simulink model "Satellite_Open_Loop_Model"  (R2018b)
settings: Solver=VariableStepAuto  StartTime=0.0  StopTime=200  RelTol=1e-3
values from neighbouring files (symbols this model uses):
  a = 0.5736    [Lab1.m]    (also in Micro_Sat_Open_Loop.m)
  J_r = 0.0004    [Lab1.m]    (also in Micro_Sat_Open_Loop.m)
  J_s = 31.38    [Lab1.m]    (also in Micro_Sat_Open_Loop.m)
  noise = 10^-9    (= 1e-09)    [Lab1.m]    (also in Micro_Sat_Open_Loop.m)
  T_d = 0.001    [Lab1.m]    (also in Micro_Sat_Open_Loop.m)
  T_e = 0.5    [Lab1.m]    (also in Micro_Sat_Open_Loop.m)
  Tc_max = 0.05    [Lab1.m]    (also in Micro_Sat_Open_Loop.m)
  To_m = 0.8    [Lab1.m]    (also in Micro_Sat_Open_Loop.m)
  w = 2.6268    [Lab1.m]    (also in Micro_Sat_Open_Loop.m)
  w_sat = wr_max*2*pi/60    (= 293.215314335)    [Micro_Sat_Open_Loop.m]
undefined symbols (not defined in the file or in its folder): sigbuilder_block
settings Model: Creator=Yavuz  LastModifiedBy=EKOCULU

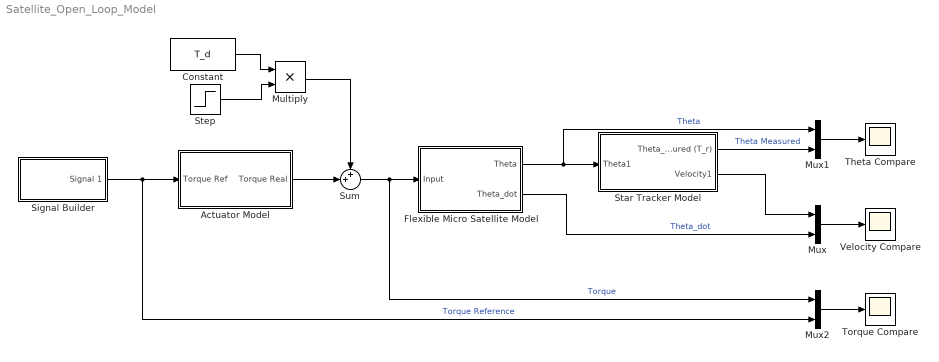
== system Satellite_Open_Loop_Model ==
  Actuator Model : Subsystem
  Constant : Constant  Value=T_d
  "Flexible Micro Satellite Model " : Subsystem
  Multiply : Product
  Mux : Mux  Inputs=2
  Mux1 : Mux  Inputs=2
  Mux2 : Mux  Inputs=2
  Signal Builder : Subsystem  Tag=STV Subsys  LoadFcn=sigbuilder_block('load');  StartFcn=sigbuilder_block('start');  StopFcn=sigbuilder_block('stop');  ClipboardFcn=sigbuilder_block('clipboard');  mask(Sigbuilder block){tuvar=[0:10]}
      mask help: Simulink:masks:SigbuilderBlock_MD
      mask init:
      | if ~strcmp(get_param(bdroot(gcbh),'SimulationStatus'),'stopped') tuvar = sigbuilder_block('maskInit'); end
      settings: CopyFcn=sigbuilder_block('copy');  DeleteFcn=sigbuilder_block('delete');  ModelCloseFcn=sigbuilder_block('modelClose');  PreSaveFcn=sigbuilder_block('preSave');  PauseFcn=sigbuilder_block('pause');  ContinueFcn=sigbuilder_block('continue');  NameChangeFcn=sigbuilder_block('namechange');  OpenFcn=sigbuilder_block('open',[6 30 1428 681.75 ]);  CloseFcn=sigbuilder_block('close');
      mask Display: plot(0, 0, 100, 100,[2, 2, 32, 32, 2], [68, 8, 8, 68, 68],[32, 2], [38, 38], [32, 19, 2],[53, 60, 44], [32, 17, 17, 2],[16, 16, 31, 31]);txt = getActiveGroup(gcbh);text(2, 100, txt,'verticalAlignment', 'top');
  Star Tracker Model : Subsystem
  Step : Step  Time=100  SampleTime=0
  Sum : Sum  Inputs=++|
  Theta Compare : Scope
  Torque Compare : Scope
  Velocity Compare : Scope
  wires:
  "Flexible Micro Satellite Model "/1(Theta) -> Star Tracker Model/1(Theta1), Mux1/1  "Theta"
  Sum/1 -> Mux2/1, "Flexible Micro Satellite Model "/1(Input)  "Torque"
  Actuator Model/1(Torque Real) -> Sum/2
  Constant/1 -> Multiply/1
  Step/1 -> Multiply/2
  Multiply/1 -> Sum/1
  "Flexible Micro Satellite Model "/2(Theta_dot) -> Mux/2  "Theta_dot"
  Mux/1 -> Velocity Compare/1
  Mux1/1 -> Theta Compare/1
  Star Tracker Model/1(Theta_measured (T_r)) -> Mux1/2  "Theta Measured"
  Mux2/1 -> Torque Compare/1
  Signal Builder/1(Signal 1) -> Mux2/2, Actuator Model/1(Torque Ref)  "Torque Reference"
  Star Tracker Model/2(Velocity1) -> Mux/1

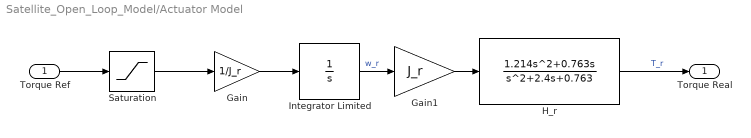
== system Satellite_Open_Loop_Model/Actuator Model ==
  Torque Ref : Inport
  Gain : Gain  Gain=1/J_r
  Gain1 : Gain  Gain=J_r
  H_r : TransferFcn  Numerator=[1.214 0.763 0]  Denominator=[1 2.4 0.763]
  Integrator Limited : Integrator  LimitOutput=on  UpperSaturationLimit=w_sat  LowerSaturationLimit=0
  Saturation : Saturate  UpperLimit=Tc_max  LowerLimit=-Tc_max
  Torque Real : Outport
  wires:
  Saturation/1 -> Gain/1
  Torque Ref/1 -> Saturation/1
  Gain1/1 -> H_r/1
  Gain/1 -> Integrator Limited/1
  H_r/1 -> Torque Real/1  "T_r"
  Integrator Limited/1 -> Gain1/1  "w_r"

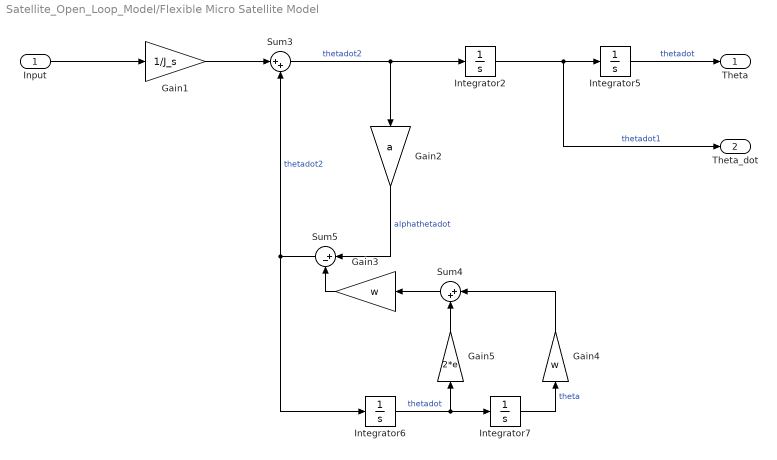
== system Satellite_Open_Loop_Model/Flexible Micro Satellite Model  ==
  Input : Inport
  Gain1 : Gain  Gain=1/J_s
  Gain2 : Gain  Gain=a
  Gain3 : Gain  Gain=w
  Gain4 : Gain  Gain=w
  Gain5 : Gain  Gain=2*e
  Integrator{2,5..7} (4 alike) : Integrator
  Sum3 : Sum  Inputs=|++
  Sum4 : Sum  Inputs=|++
  Sum5 : Sum  Inputs=|+-
  Theta : Outport
  Theta_dot : Outport  Port=2
  wires:
  Integrator5/1 -> Theta/1  "thetadot"
  Input/1 -> Gain1/1
  Gain5/1 -> Sum4/2
  Gain3/1 -> Sum5/2
  Integrator2/1 -> Theta_dot/1, Integrator5/1  "thetadot1"
  Gain2/1 -> Sum5/1  "alphathetadot"
  Integrator7/1 -> Gain4/1  "theta"
  Gain1/1 -> Sum3/1
  Sum5/1 -> Integrator6/1, Sum3/2  "thetadot2"
  Integrator6/1 -> Gain5/1, Integrator7/1  "thetadot"
  Sum3/1 -> Gain2/1, Integrator2/1  "thetadot2"
  Sum4/1 -> Gain3/1
  Gain4/1 -> Sum4/1

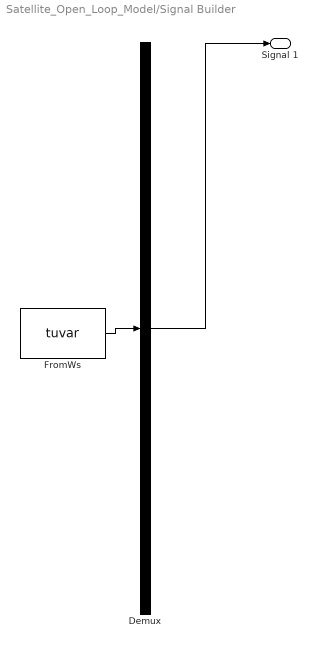
== system Satellite_Open_Loop_Model/Signal Builder ==
  Demux : Demux  Tag=STV Demux  Outputs=1
  FromWs : FromWorkspace  Tag=STV FromWs  VariableName=tuvar  SampleTime=0
      SigBuilderData=|
      | common.afterFinalStr = 'Extrapolate'
      | common.sampleTime = 0
      | dataSet.timeRange = [0 200]
      | dataSet.name = 'Group 1'
      | sbobj.Groups.Name = 'Group 1'
      | sbobj.Groups.Signals.Name = 'Signal 1'
      | sbobj.Groups.Signals.XData = [0 20 20 80 80 140 140 200]
      | sbobj.Groups.Signals.YData = [0 0 0.003 0.003 -0.003 -0.003 0 0]
      | sbobj.Groups.TimeRange = [0 200]
  Signal 1 : Outport  Tag=STV Outport
  wires:
  Demux/1 -> Signal 1/1
  FromWs/1 -> Demux/1

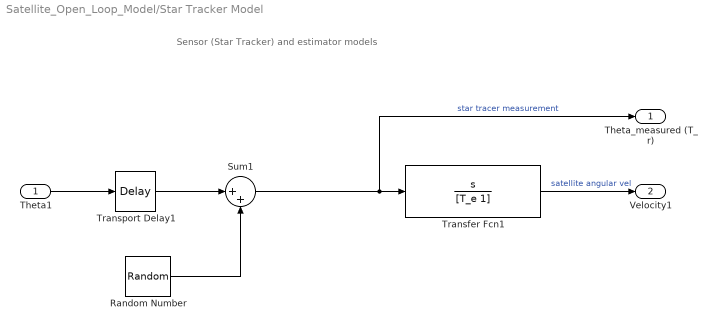
== system Satellite_Open_Loop_Model/Star Tracker Model ==
  note: Sensor (Star Tracker) and estimator models
  Theta1 : Inport
  Random Number : RandomNumber  Variance=noise  SampleTime=0.1
  Sum1 : Sum  Inputs=|++
  Transfer Fcn1 : TransferFcn  Numerator=[1 0]  Denominator=[T_e 1]
  Transport Delay1 : TransportDelay  DelayTime=To_m
  Theta_measured (T_r) : Outport
  Velocity1 : Outport  Port=2
  wires:
  Sum1/1 -> Theta_measured (T_r)/1, Transfer Fcn1/1  "star tracer measurement"
  Theta1/1 -> Transport Delay1/1
  Random Number/1 -> Sum1/2
  Transport Delay1/1 -> Sum1/1
  Transfer Fcn1/1 -> Velocity1/1  "satellite angular vel"
